simulink model "task3"  (R2019b)
settings: Solver=FixedStepDiscrete  StartTime=0.0  StopTime=20.0  FixedStep=0.01  RelTol=1e-3
settings Model: EnablePacing=on  PacingRate=0.250000  Creator=linesLK  LastModifiedBy=linesLK

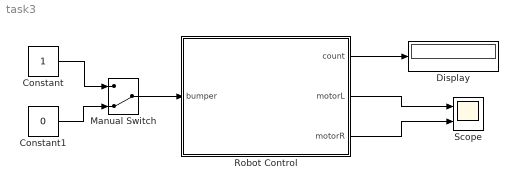
== system task3 ==
  Constant : Constant
  Constant1 : Constant  Value=0
  Display : Display
  Manual Switch : ManualSwitch  CurrentSetting=0
  Robot Control : Stateflow chart  BlockKeywords=__PRM__SERIALIZED__DATA__:Stateflow Chart,Stateflow Diagram  TreatAsAtomicUnit=on
  Scope : Scope  NumInputPorts=2
  wires:
  Robot Control/1(count) -> Display/1
  Manual Switch/1 -> Robot Control/1(bumper)
  Constant/1 -> Manual Switch/1
  Constant1/1 -> Manual Switch/2
  Robot Control/2(motorL) -> Scope/1
  Robot Control/3(motorR) -> Scope/2

== stateflow chart task3/Robot Control ==
  state reverse
    entry: motorL = -1;
    entry: motorR = -1;
  state forwards
    entry: motorL = 1;
    entry: motorR = 1;
  state rotate
    entry: motorL = rand(1);
    entry: motorR = rand(1);
  forwards -> reverse : [bumper == 0]{count = count + 1;}
  reverse -> rotate : [after(2,sec)]
  (default) -> forwards
  rotate -> forwards : [after(2,sec)]
  data: count output double =0; bumper input double; motorL output double; motorR output double
